simulink model "udptest"  (Simulink 7.5)
settings: Solver=FixedStepDiscrete  SolverMode=SingleTasking  StartTime=0.0  StopTime=5  FixedStep=1  RelTol=1e-3
libraries: udp_library x3
settings Model: Creator=paul  LastModifiedBy=paul.liu
settings OptimizationCC: OptimizeModelRefInitCode=on  LifeSpan=1
settings DebuggingCC: InheritedTsInSrcMsg=none  FcnCallInpInsideContextMsg=Enable All
settings RTWCC: SystemTargetFile=ert.tlc  TemplateMakefile=ert_default_tmf  Description=Real-Time Workshop Embedded Coder  ProcessScript=ert_make_rtw_hook
settings CodeAppCC: IgnoreCustomStorageClasses=off
settings ERTTargetCC: MultiwordLength=2048  GenerateSampleERTMain=on  SupportNonInlinedSFcns=on  ERTCustomFileTemplate=example_file_process.tlc  ConvertIfToSwitch=off

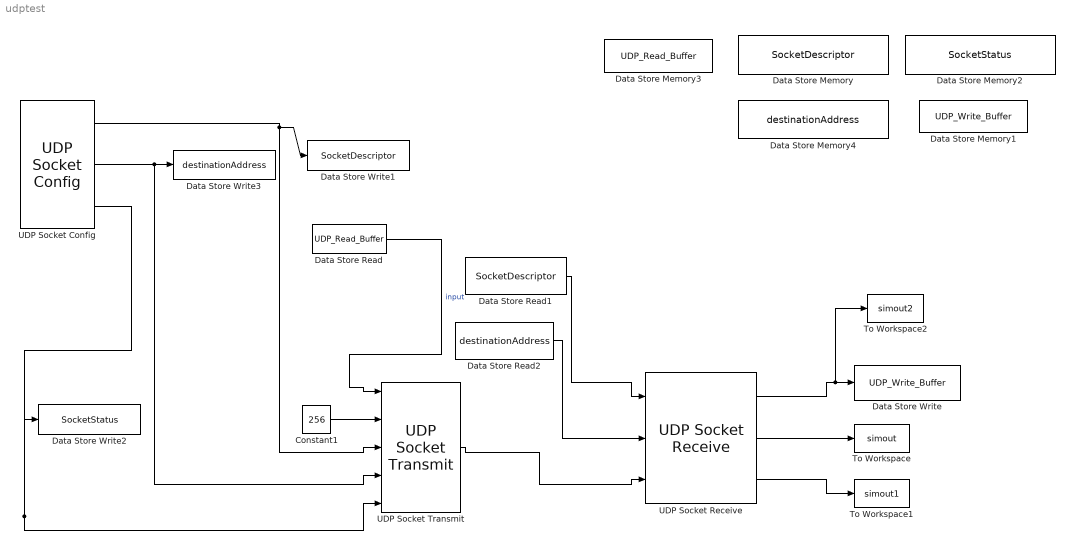
== system udptest ==
  Constant1 : Constant  Value=256  OutDataTypeMode=uint32  OutDataTypeStr=uint32
  Data Store Memory : DataStoreMemory  DataStoreName=SocketDescriptor  ReadBeforeWriteMsg=warning  WriteAfterWriteMsg=warning  WriteAfterReadMsg=warning  DataType=uint32  OutDataType=fixdt(1, 16)  OutScaling=2^0  OutDataTypeStr=uint32
  Data Store Memory1 : DataStoreMemory  DataStoreName=UDP_Write_Buffer  ReadBeforeWriteMsg=warning  WriteAfterWriteMsg=warning  WriteAfterReadMsg=warning  InitialValue=[0 0 0 0 0 0 0 0 0 0 0 0 0 0 0 0 0 0 0 0 0 0 0 0 0 0 0 0 0 0 0 0 0 0 0 0 0 0 0 0 0 0 0 0 0 0 0 0 0 0 0 0 0 0 0 0 0 0 0 0 0 0 0 0]  DataType=uint32  OutDataTypeStr=uint32
  Data Store Memory2 : DataStoreMemory  DataStoreName=SocketStatus  ReadBeforeWriteMsg=warning  WriteAfterWriteMsg=warning  WriteAfterReadMsg=warning  DataType=int32  OutDataType=fixdt(1, 16)  OutScaling=2^0  OutDataTypeStr=int32
  Data Store Memory3 : DataStoreMemory  DataStoreName=UDP_Read_Buffer  ReadBeforeWriteMsg=warning  WriteAfterWriteMsg=warning  WriteAfterReadMsg=warning  InitialValue=[1 2 3 4 5 6 7 8 9 0 1 2 3 4 5 6 7 8 9 0 1 2 3 4 5 6 7 8 9 0 1 2 3 4 5 6 7 8 9 0 1 2 3 4 5 6 7 8 9 0 1 2 3 4 5 6 7 8 9 0 1 2 3 4]  DataType=uint32  OutDataTypeStr=uint32
  Data Store Memory4 : DataStoreMemory  DataStoreName=destinationAddress  ReadBeforeWriteMsg=warning  WriteAfterWriteMsg=warning  WriteAfterReadMsg=warning  DataType=uint32  OutDataType=fixdt(1, 16)  OutScaling=2^0  OutDataTypeStr=uint32
  Data Store Read : DataStoreRead  DataStoreName=UDP_Read_Buffer  SampleTime=-1
  Data Store Read1 : DataStoreRead  DataStoreName=SocketDescriptor  SampleTime=0
  Data Store Read2 : DataStoreRead  DataStoreName=destinationAddress  SampleTime=0
  Data Store Write : DataStoreWrite  DataStoreName=UDP_Write_Buffer  SampleTime=-1
  Data Store Write1 : DataStoreWrite  DataStoreName=SocketDescriptor  SampleTime=-1
  Data Store Write2 : DataStoreWrite  DataStoreName=SocketStatus  SampleTime=-1
  Data Store Write3 : DataStoreWrite  DataStoreName=destinationAddress  SampleTime=-1
  To Workspace : ToWorkspace  VariableName=simout  SampleTime=-1  SaveFormat=Structure
  To Workspace1 : ToWorkspace  VariableName=simout1  SampleTime=-1  SaveFormat=Structure
  To Workspace2 : ToWorkspace  VariableName=simout2  SampleTime=-1  SaveFormat=Structure
  UDP Socket Config : udp_library/UDP Socket Config  SystemSampleTime=-1  server_ip='127.0.0.1'  server_port=1002  client_ip='127.0.0.1'  client_port=1001
      link override UDP Socket Configuration: server_ip='127.0.0.1'  server_port=1002  client_ip='127.0.0.1'  client_port=1001
      settings: AttributesFormatString=Ver 1.0
  UDP Socket Receive : udp_library/UDP Socket Receive  SystemSampleTime=-1
      settings: AttributesFormatString=Ver 1.0
  UDP Socket Transmit : udp_library/UDP Socket Transmit  SystemSampleTime=-1
      settings: AttributesFormatString=Ver 1.0
  wires:
  Data Store Read/1 -> UDP Socket Transmit/1  "input"
  UDP Socket Config/1 -> Data Store Write1/1, UDP Socket Transmit/3
  UDP Socket Config/3 -> Data Store Write2/1, UDP Socket Transmit/5
  UDP Socket Config/2 -> Data Store Write3/1, UDP Socket Transmit/4
  Constant1/1 -> UDP Socket Transmit/2
  UDP Socket Transmit/1 -> UDP Socket Receive/3
  Data Store Read1/1 -> UDP Socket Receive/1
  Data Store Read2/1 -> UDP Socket Receive/2
  UDP Socket Receive/1 -> Data Store Write/1, To Workspace2/1
  UDP Socket Receive/3 -> To Workspace1/1
  UDP Socket Receive/2 -> To Workspace/1
